simulink model "Ex4_model"  (R2024b)
settings: Solver=VariableStepAuto  StartTime=0.0  StopTime=1  RelTol=1e-3
values from neighbouring files (symbols this model uses):
  A = [0, 1; 0, -10]    [Ex1_script.m]    (also in Ex3_script.m = [0, 1; -2, -40]; Ex4_script.m = [0,1; 0,-20])
  B = [0; 120]    [Ex1_script.m]    (also in Ex3_script.m = [0; 40]; Ex4_script.m = [0; 60])
  C = [1, 0]    [Ex1_script.m]    (also in Ex3_script.m; Ex4_script.m)
  D = 0    [Ex1_script.m]    (also in Ex3_script.m; Ex4_script.m)
  den_hp = [1, 2*del*wc, wc^2]    [Ex4_script.m]
  den_tf = [1, -Ar(end,:)]    [Ex4_script.m]
  K = Kr    [Ex2_script.m]    (also in Ex3_script.m = Ke(2:3); Ex4_script.m = Ke(4:5))
  num_hp = [wc^2, 0]    [Ex4_script.m]
  num_tf = flip(Ktf)    [Ex4_script.m]
settings Model: Creator=pries  LastModifiedBy=pries

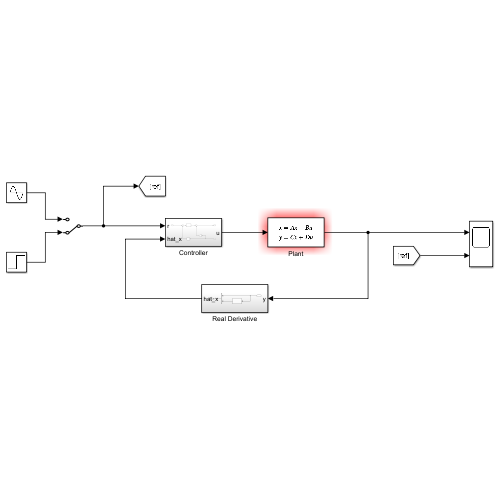
[thumbnail: Simulink's stored preview of the top-level diagram]
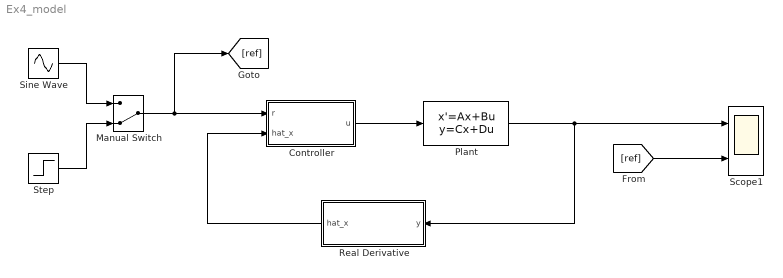
== system Ex4_model ==
  Controller : Subsystem
  Manual Switch : ManualSwitch  CurrentSetting=0
  Plant : StateSpace  A=A  B=B  C=C  D=D  InitialCondition=0
  Real Derivative : Subsystem
  Scope1 : Scope  NumInputPorts=2
  Sine Wave : Sin  Frequency=6  SampleTime=0
  Step : Step  Time=0  SampleTime=0
  wires:
  Controller/1(u) -> Plant/1
  Plant/1 -> Real Derivative/1(y), Scope1/1
  Real Derivative/1(hat_x) -> Controller/2(hat_x)
  [ref] -> Scope1/2
  Manual Switch/1 -> [ref], Controller/1(r)
  Sine Wave/1 -> Manual Switch/1
  Step/1 -> Manual Switch/2

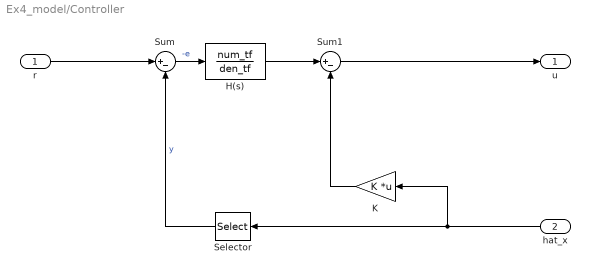
== system Ex4_model/Controller ==
  r : Inport
  hat_x : Inport  Port=2
  H(s) : TransferFcn  Numerator=num_tf  Denominator=den_tf
  K : Gain  Gain=K  Multiplication=Matrix(K*u)
  Selector : Selector  InputPortWidth=2  IndexOptions=Index vector (dialog)  Indices=1  OutputSizes=1
  Sum : Sum  Inputs=|+-
  Sum1 : Sum  Inputs=|+-
  u : Outport
  wires:
  r/1 -> Sum/1
  Selector/1 -> Sum/2  "y"
  hat_x/1 -> Selector/1, K/1
  Sum/1 -> H(s)/1  "-e"
  H(s)/1 -> Sum1/1
  K/1 -> Sum1/2
  Sum1/1 -> u/1

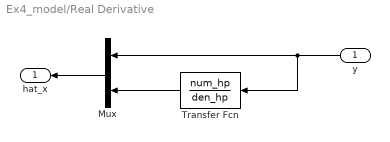
== system Ex4_model/Real Derivative ==
  y : Inport
  Mux : Mux  Inputs=2
  Transfer Fcn : TransferFcn  Numerator=num_hp  Denominator=den_hp
  hat_x : Outport
  wires:
  Mux/1 -> hat_x/1
  y/1 -> Transfer Fcn/1, Mux/1
  Transfer Fcn/1 -> Mux/2
